simulink model "debugLength"  (R2024b)
settings: Solver=FixedStepDiscrete  StartTime=0.0  StopTime=10  RelTol=1e-3  EnableMultiTasking=on
libraries: simulink x3
settings Model: Creator=The MathWorks, Inc.  LastModifiedBy=kev
settings SolverCC: AlgebraicLoopSolver=TrustRegion
settings DataIOCC: LimitDataPoints=on  SaveFormat=StructureWithTime
settings OptimizationCC: ExpressionDepthLimit=2147483647  LifeSpan=inf
settings DebuggingCC: SolverPrmCheckMsg=warning  FcnCallInpInsideContextMsg=warning  UnconnectedInputMsg=warning  UnconnectedOutputMsg=warning  UnconnectedLineMsg=warning  AllowSymbolicDim=off  StateNameClashWarn=warning  SFUnexpectedBacktrackingDiag=warning  SFNoUnconditionalDefaultTransitionDiag=warning  SFExecutionAtInitializationDiag=none  ArithmeticOperatorsInVariantConditions=warning
settings HardwareCC: ProdBitPerPointer=32  ProdBitPerSizeT=32  ProdBitPerPtrDiffT=32  ProdLargestAtomicFloat=None  ProdIntDivRoundTo=Undefined  ProdEndianess=Unspecified  ProdWordSize=32  ProdHWDeviceType=32-bit Generic
settings ModelReferenceCC: EnableRefExpFcnMdlSchedulingChecks=on  PropagateSignalLabelsOutOfModel=off
settings SFSimCC: SimUseLocalCustomCode=off  SimParseCustomCode=off  CustomCodeUndefinedFunction=UseInterfaceOnly
settings RTWCC: RTWUseLocalCustomCode=off  GPUComputeCapability=3.5  DLArmComputeVersion=19.05
settings CodeAppCC: StateflowObjectComments=on
settings GRTTargetCC: TargetLangStandard=C89/C90 (ANSI)  CombineOutputUpdateFcns=off  GRTInterface=on
settings ConfigComp: CovMetricSettings=dw  CovSaveCumulativeToWorkspaceVar=on  CovSaveSingleToWorkspaceVar=on  CovExternalEMLEnable=off

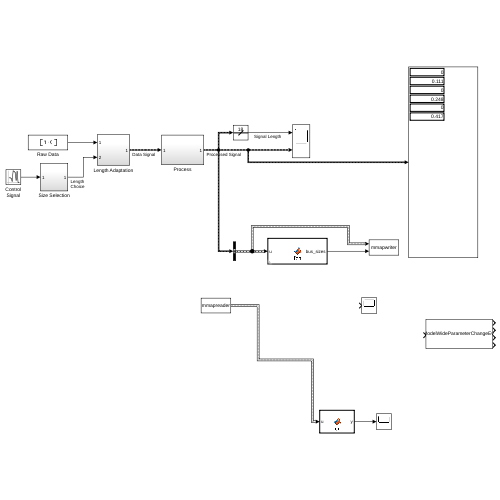
[thumbnail: Simulink's stored preview of the top-level diagram]
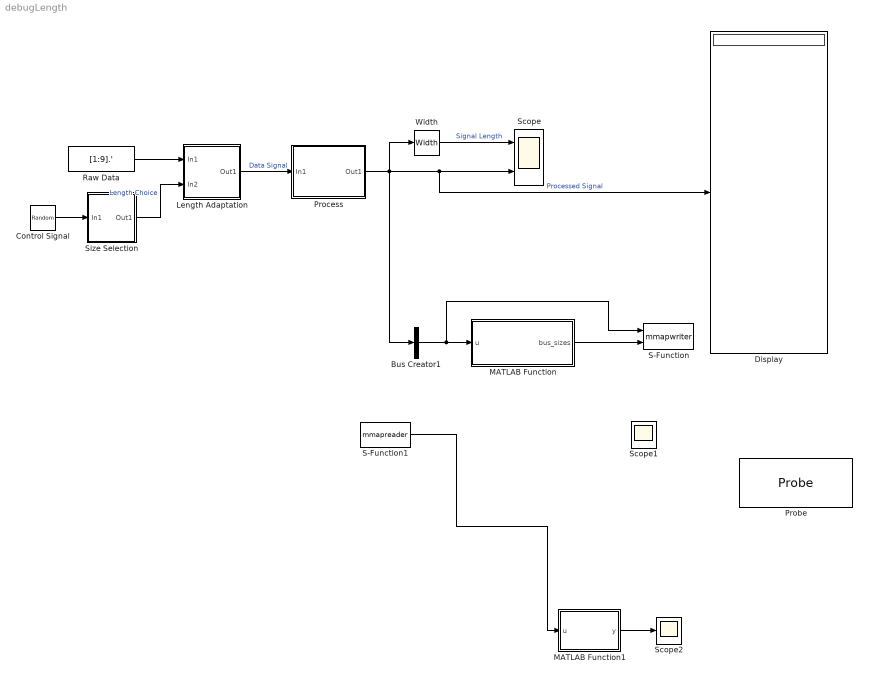
== system debugLength ==
  Bus Creator1 : BusCreator  Inputs=1  OutDataTypeStr=Bus: NewBus  NonVirtualBus=on
      settings: InheritFromInputs=off
  Control Signal : RandomNumber  Variance=0.5  SampleTime=0.1
  Display : Display
  Length Adaptation : Subsystem
  MATLAB Function : MATLAB Function  TreatAsAtomicUnit=on
  MATLAB Function1 : MATLAB Function  TreatAsAtomicUnit=on
  Probe : Probe  ProbeSignalDimensions=on
  Process : Subsystem
  Raw Data : Constant  Value=[1:9].'
  S-Function : S-Function  FunctionName=mmapwriter  Parameters=NewBus, 'Testing'  SFunctionDeploymentMode=off  EnableBusSupport=off
  S-Function1 : S-Function  FunctionName=mmapreader  Parameters='Testing', NewBus  SFunctionDeploymentMode=off  EnableBusSupport=off
  Scope : Scope  NumInputPorts=2
  Scope1 : Scope
  Scope2 : Scope
  Size Selection : Subsystem
  Width : Width  DataType=uint8
  wires:
  Length Adaptation/1(Out1) -> Process/1(In1)  "Data Signal"
  Width/1 -> Scope/1  "Signal Length"
  Size Selection/1(Out1) -> Length Adaptation/2(In2)  "Length Choice"
  Raw Data/1 -> Length Adaptation/1(In1)
  Process/1(Out1) -> Display/1, Scope/2, Bus Creator1/1, Width/1  "Processed Signal"
  Control Signal/1 -> Size Selection/1(In1)
  MATLAB Function/1(bus_sizes) -> S-Function/2
  Bus Creator1/1 -> MATLAB Function/1("u "), S-Function/1
  S-Function1/1 -> MATLAB Function1/1(u)
  MATLAB Function1/1(y) -> Scope2/1

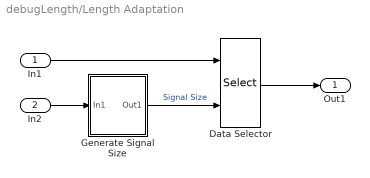
== system debugLength/Length Adaptation ==
  In1 : Inport
  In2 : Inport  Port=2
  Data Selector : Selector  InputPortWidth=9  IndexOptions=Starting and ending indices (port)  Indices=[1 3]  OutputSizes=32
  Generate Signal Size : Subsystem
  Out1 : Outport  VectorParamsAs1DForOutWhenUnconnected=off
  wires:
  Data Selector/1 -> Out1/1
  In1/1 -> Data Selector/1
  In2/1 -> Generate Signal Size/1(In1)
  Generate Signal Size/1(Out1) -> Data Selector/2  "Signal Size"

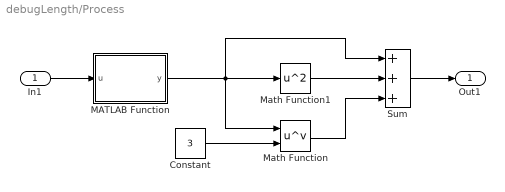
== system debugLength/Process ==
  In1 : Inport
      settings: VarSizeSig=Yes
  Constant : Constant  Value=3
  MATLAB Function : MATLAB Function  TreatAsAtomicUnit=on
  Math Function : Math  Operator=pow  SignedPower=on
  Math Function1 : Math  Operator=square  SignedPower=on
  Sum : Sum  Inputs=+++
  Out1 : Outport  VectorParamsAs1DForOutWhenUnconnected=off
  wires:
  In1/1 -> MATLAB Function/1(u)
  MATLAB Function/1(y) -> Math Function/1, Math Function1/1, Sum/1
  Math Function1/1 -> Sum/2
  Sum/1 -> Out1/1
  Constant/1 -> Math Function/2
  Math Function/1 -> Sum/3

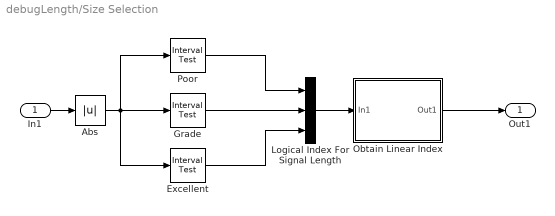
== system debugLength/Size Selection ==
  In1 : Inport
  Abs : Abs  SaturateOnIntegerOverflow=off
  Excellent : simulink/Logic and Bit Operations/Interval Test  IntervalClosedRight=off  uplimit=inf  IntervalClosedLeft=on  lowlimit=0.50  OutDataTypeStr=uint8
  Grade : simulink/Logic and Bit Operations/Interval Test  IntervalClosedRight=off  uplimit=0.50  IntervalClosedLeft=on  lowlimit=0.25  OutDataTypeStr=uint8
  Logical Index For Signal Length : Concatenate  NumInputs=3
  Obtain Linear Index : Subsystem
  Poor : simulink/Logic and Bit Operations/Interval Test  IntervalClosedRight=off  uplimit=0.25  IntervalClosedLeft=on  lowlimit=0.0  OutDataTypeStr=uint8
  Out1 : Outport  VectorParamsAs1DForOutWhenUnconnected=off
  wires:
  Obtain Linear Index/1(Out1) -> Out1/1
  Grade/1 -> Logical Index For Signal Length/2
  Excellent/1 -> Logical Index For Signal Length/3
  Poor/1 -> Logical Index For Signal Length/1
  Logical Index For Signal Length/1 -> Obtain Linear Index/1(In1)
  Abs/1 -> Grade/1, Poor/1, Excellent/1
  In1/1 -> Abs/1

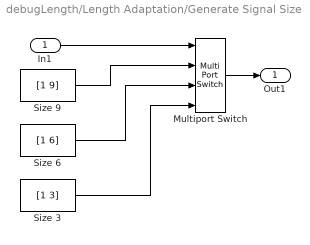
== system debugLength/Length Adaptation/Generate Signal Size ==
  In1 : Inport
  Multiport Switch : MultiPortSwitch  SaturateOnIntegerOverflow=off  InputSameDT=off
  Size 3 : Constant  Value=[1 3]
  Size 6 : Constant  Value=[1 6]
  Size 9 : Constant  Value=[1 9]
  Out1 : Outport  VectorParamsAs1DForOutWhenUnconnected=off
  wires:
  Size 3/1 -> Multiport Switch/4
  Size 6/1 -> Multiport Switch/3
  Size 9/1 -> Multiport Switch/2
  In1/1 -> Multiport Switch/1
  Multiport Switch/1 -> Out1/1

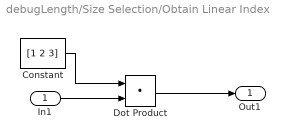
== system debugLength/Size Selection/Obtain Linear Index ==
  In1 : Inport
  Constant : Constant  Value=[1 2 3]
  Dot Product : DotProduct  InputSameDT=off  OutDataTypeStr=Inherit: Inherit via internal rule
  Out1 : Outport  VectorParamsAs1DForOutWhenUnconnected=off
  wires:
  In1/1 -> Dot Product/2
  Dot Product/1 -> Out1/1
  Constant/1 -> Dot Product/1

== matlab function debugLength/Process/MATLAB Function ==
  data: u input size=9; y output size=18
function y = fcn(u)
%#codegen
%
% Insert zeros between elements

sizeU = length(u);
y     = zeros(2*sizeU,1);
for i=1:2*sizeU
    if(mod(i,2))
        y(i)=0; 
    else
        y(i)=u(i/2)/10;
    end
end

== matlab function debugLength/MATLAB Function1 ==
  data: u input; y output
function y = fcn(u)
    y = u.a(1);
end

== matlab function debugLength/MATLAB Function ==
  data: u input; bus_sizes output int32
function bus_sizes   = fcn(u)
    flat_dims = zeros(getLen(u), 2, 'int32');
    counter = ones(1);
    [flat_dims, counter] = getDims(u, flat_dims, counter);
    bus_sizes = flat_dims;
    %disp(flat_dims);
end

function len = getLen(bus)
    fields = fieldnames(bus);
    len = 0;
    for iF = 1:numel(fields)
        field = fields{iF};
        if isfield(bus, field)
            value = bus.(field);
            if isa(value, 'struct')
                len = len + getLen(value);
            else
                len = len + 1;
            end
        end
    end
end

function [flat_dims, counter] = getDims(bus, flat_dims, counter)
    fields = fieldnames(bus);
    for iF = 1:numel(fields)
        field = fields{iF};
        if isfield(bus, field)
            value = bus.(field);
            if isa(value, 'struct')
                [flat_dims, counter] = getDims(value, flat_dims, counter);
            else
                flat_dims(counter(1), :) = size(value);
                counter(1) = counter(1) + 1;
            end
        end
    end
end
